simulink model "control"  (R2020a)
settings: Solver=FixedStepDiscrete  StartTime=0.0  StopTime=1  FixedStep=0.0005  RelTol=1e-3  EnableMultiTasking=on
undefined symbols (not defined in the file): acc_calmax1, acc_calmax2, acc_calmin1, acc_calmin2, akemancanshu, bre, bre_calmax, bre_calmin, ecucoder_acal, I_AN01_5K1, I_AN03_5V, I_AN04_5V, kd, ki, kp, leftmax, O_SW06_HS1A, rightmax, T_add, T_del, tiaoshi, zhiling
libraries: ec5744lib x252, canmsglib x92, simulink x5
(part 7 of 9)

== system control/Subsystem/run/analog_input/无人意图转译/无人/Subsystem1/Desired ==
  此处输入感知的期望整车纵向速度 : Inport
  输入整车加速度测量值1 : Inport  Port=2
  输入整车车速测量值1 : Inport  Port=3
  Data Store Read3 : DataStoreRead  DataStoreName=match_model
  Data Store Write : DataStoreWrite  Commented=on  DataStoreName=acc
  MATLAB Function : MATLAB Function  TreatAsAtomicUnit=on
  MATLAB Function1 : MATLAB Function  Commented=on  TreatAsAtomicUnit=on
  MATLAB Function2 : MATLAB Function  TreatAsAtomicUnit=on
  Subsystem : Subsystem
  Subsystem1 : Subsystem
  ddotx1d输入1 : Outport
  dotx1d输入 : Outport  Port=2
  x1d输入 : Outport  Port=3
  输入整车加速度测量值x2 : Outport  Port=4
  输入整车车速测量值x1 : Outport  Port=5
  wires:
  此处输入感知的期望整车纵向速度/1 -> MATLAB Function2/7(v1), Subsystem1/1(y), MATLAB Function/1(u)
  输入整车加速度测量值1/1 -> 输入整车加速度测量值x2/1
  MATLAB Function1/1(y) -> ddotx1d输入1/1
  MATLAB Function/1(y) -> MATLAB Function2/1(u1), Subsystem/1(y)
  MATLAB Function2/1(y) -> MATLAB Function1/1(u), dotx1d输入/1, Data Store Write/1
  Subsystem/1(u2) -> MATLAB Function2/2(u2)
  Subsystem/2(u3) -> MATLAB Function2/3(u3)
  Subsystem/3(u4) -> MATLAB Function2/4(u4)
  Subsystem/4(u5) -> MATLAB Function2/5(u5)
  输入整车车速测量值1/1 -> 输入整车车速测量值x1/1
  Data Store Read3/1 -> MATLAB Function2/6(model)
  Subsystem1/1(u2) -> MATLAB Function2/8(v2)
  Subsystem1/2(u3) -> MATLAB Function2/9(v3)
  Subsystem1/3(u4) -> MATLAB Function2/10(v4)
  Subsystem1/4(u5) -> MATLAB Function2/11(v5)
  MATLAB Function2/2(V) -> x1d输入/1

== system control/Subsystem/run/analog_input/无人意图转译/无人/Subsystem1/Subsystem ==
  note: 反馈系数，得调一下
  期望加速度（负值） : Inport
  x1d输入 : Inport  Port=2
  输入整车车速测量值x1 : Inport  Port=3
  Abs : Abs
  Abs1 : Abs
  MATLAB Function : MATLAB Function  TreatAsAtomicUnit=on
  Product : Product
  Sum : Sum  Inputs=|++
  pid_function : Subsystem
  整车质量 : Constant  Value=246
  总制动力 : Outport
  wires:
  期望加速度（负值）/1 -> pid_function/2(期望加速度（负值）), Abs/1
  Abs/1 -> Product/2
  整车质量/1 -> Product/1
  Product/1 -> Sum/1
  [A] -> pid_function/1(u)
  pid_function/1(output) -> Abs1/1
  Abs1/1 -> Sum/2
  Sum/1 -> MATLAB Function/1(u)
  输入整车车速测量值x1/1 -> MATLAB Function/2(v)
  x1d输入/1 -> MATLAB Function/3(vd)
  MATLAB Function/1(y) -> 总制动力/1

== system control/Subsystem/run/analog_input/无人意图转译/无人/Subsystem1/计算四轮各自制动力 ==
  u : Inport
  Data Store Read : DataStoreRead  DataStoreName=M_expire
  MATLAB Function : MATLAB Function  TreatAsAtomicUnit=on
  输出左前的制动力 : Outport
  输出右前的制动力2 : Outport  Port=2
  输出左后轮的制动力3 : Outport  Port=3
  输出右后轮的制动力1 : Outport  Port=4
  wires:
  u/1 -> MATLAB Function/1(u)
  MATLAB Function/1(y1) -> 输出左前的制动力/1
  MATLAB Function/2(y2) -> 输出右前的制动力2/1
  MATLAB Function/3(y3) -> 输出左后轮的制动力3/1
  MATLAB Function/4(y4) -> 输出右后轮的制动力1/1
  Data Store Read/1 -> MATLAB Function/2(deltaM)

== system control/Subsystem/run/ctrl/Subsystem1/control_strategy/Subsystem/Rules ==
  as : Inport
  am : Inport  Port=2
  ab : Inport  Port=3
  bnb : Inport  Port=4
  bns : Inport  Port=5
  bo : Inport  Port=6
  bps : Inport  Port=7
  bpb : Inport  Port=8
  DNB : MinMax  Function=max
  DNS : MinMax  Function=max  Inputs=3
  DO : MinMax  Function=max  Inputs=3
  DPB : MinMax  Function=max  Inputs=4
  DPS : MinMax  Function=max  Inputs=4
  Min(AB,BNB) : MinMax  Inputs=2
  Min(AB,BNS) : MinMax  Inputs=2
  Min(AB,BO) : MinMax  Inputs=2
  Min(AB,BPB) : MinMax  Inputs=2
  Min(AB,BPS) : MinMax  Inputs=2
  Min(AM,BNB) : MinMax  Inputs=2
  Min(AM,BNS) : MinMax  Inputs=2
  Min(AM,BO) : MinMax  Inputs=2
  Min(AM,BPB) : MinMax  Inputs=2
  Min(AM,BPS) : MinMax  Inputs=2
  Min(AS,BNB) : MinMax  Inputs=2
  Min(AS,BNS) : MinMax  Inputs=2
  Min(AS,BO) : MinMax  Inputs=2
  Min(AS,BPB) : MinMax  Inputs=2
  Min(AS,BPS) : MinMax  Inputs=2
  dnb : Outport  VectorParamsAs1DForOutWhenUnconnected=off
  dns : Outport  Port=2  VectorParamsAs1DForOutWhenUnconnected=off
  do : Outport  Port=3  VectorParamsAs1DForOutWhenUnconnected=off
  dps : Outport  Port=4  VectorParamsAs1DForOutWhenUnconnected=off
  dpb : Outport  Port=5  VectorParamsAs1DForOutWhenUnconnected=off
  wires:
  Min(AS,BNS)/1 -> DNS/1
  Min(AB,BNB)/1 -> DNS/3
  bps/1 -> Min(AB,BPS)/2, Min(AM,BPS)/2, Min(AS,BPS)/2
  bo/1 -> Min(AB,BO)/2, Min(AM,BO)/2, Min(AS,BO)/2
  bpb/1 -> Min(AB,BPB)/2, Min(AM,BPB)/2, Min(AS,BPB)/2
  as/1 -> Min(AS,BPB)/1, Min(AS,BPS)/1, Min(AS,BO)/1, Min(AS,BNS)/1, Min(AS,BNB)/1
  Min(AS,BNB)/1 -> DNB/1
  Min(AS,BPB)/1 -> DPB/1
  bns/1 -> Min(AB,BNS)/2, Min(AM,BNS)/2, Min(AS,BNS)/2
  Min(AB,BNS)/1 -> DO/3
  ab/1 -> Min(AB,BPB)/1, Min(AB,BPS)/1, Min(AB,BO)/1, Min(AB,BNS)/1, Min(AB,BNB)/1
  bnb/1 -> Min(AM,BNB)/2, Min(AS,BNB)/2, Min(AB,BNB)/2
  Min(AM,BO)/1 -> DPS/3
  am/1 -> Min(AM,BPB)/1, Min(AM,BPS)/1, Min(AM,BO)/1, Min(AM,BNS)/1, Min(AM,BNB)/1
  Min(AB,BPB)/1 -> DPB/3
  Min(AM,BNB)/1 -> DNS/2
  Min(AS,BPS)/1 -> DPS/1
  Min(AM,BPS)/1 -> DPS/2
  Min(AM,BNS)/1 -> DO/2
  Min(AB,BO)/1 -> DPS/4
  Min(AS,BO)/1 -> DO/1
  Min(AM,BPB)/1 -> DPB/2
  Min(AB,BPS)/1 -> DPB/4
  DO/1 -> do/1
  DNB/1 -> dnb/1
  DNS/1 -> dns/1
  DPS/1 -> dps/1
  DPB/1 -> dpb/1

== system control/Subsystem/run/ctrl/Subsystem1/control_strategy/差速/差速 ==
  note: *待更改
  Data Store Read : DataStoreRead  DataStoreName=workstation_steering
  Data Store Read1 : DataStoreRead  DataStoreName=V_Kalman
  Data Store Read2 : DataStoreRead  DataStoreName=A_cexiang
  Data Store Read3 : DataStoreRead  DataStoreName=ACC_Z
  Data Store Read4 : DataStoreRead  Commented=on  DataStoreName=dianji_velcoity_zuoqian
  Data Store Read5 : DataStoreRead  Commented=on  DataStoreName=dianji_velcoity_youqian
  Data Store Read6 : DataStoreRead  Commented=on  DataStoreName=dianji_velcoity_zuohou
  Data Store Read7 : DataStoreRead  Commented=on  DataStoreName=dianji_velcoity_youhou
  Data Store Read8 : DataStoreRead  DataStoreName=workstation_steering
  Data Store Write1 : DataStoreWrite  Commented=on  DataStoreName=Vzuoqian
  Data Store Write2 : DataStoreWrite  Commented=on  DataStoreName=Vyouqian
  Data Store Write3 : DataStoreWrite  Commented=on  DataStoreName=Vzuohou
  Data Store Write4 : DataStoreWrite  Commented=on  DataStoreName=Vyouhou
  LQR差速 : MATLAB Function  TreatAsAtomicUnit=on
  MATLAB Function : MATLAB Function  TreatAsAtomicUnit=on
  Product : Product
  Sum : Sum  Inputs=|+-
  pid : MATLAB Function  Commented=on  TreatAsAtomicUnit=on
  pid1 : MATLAB Function  Commented=on  TreatAsAtomicUnit=on
  pid2 : MATLAB Function  Commented=on  TreatAsAtomicUnit=on
  pid3 : MATLAB Function  Commented=on  TreatAsAtomicUnit=on
  期望横摆力矩计算 : MATLAB Function  TreatAsAtomicUnit=on
  转动惯量 : Constant  Value=145
  阿克曼转向 : MATLAB Function  Commented=on  TreatAsAtomicUnit=on
  M : Outport
  wires:
  Product/1 -> Sum/2
  MATLAB Function/1(y) -> 期望横摆力矩计算/1(delta)
  期望横摆力矩计算/1(Mz) -> Sum/1
  Data Store Read1/1 -> 阿克曼转向/1(v), 期望横摆力矩计算/2(Vx)
  转动惯量/1 -> Product/1, LQR差速/3(J)
  Data Store Read/1 -> MATLAB Function/1(u)
  Sum/1 -> LQR差速/1(yaw_error)
  Data Store Read3/1 -> Product/2, LQR差速/2(yaw_rate)
  阿克曼转向/3(wrl) -> Data Store Write3/1
  Data Store Read4/1 -> pid/1(v)
  Data Store Read7/1 -> pid3/1(v)
  阿克曼转向/2(wfr) -> Data Store Write2/1
  Data Store Read5/1 -> pid1/1(v)
  Data Store Read2/1 -> 阿克曼转向/2(a), 期望横摆力矩计算/3(ax)
  阿克曼转向/1(wfl) -> Data Store Write1/1
  Data Store Read6/1 -> pid2/1(v)
  阿克曼转向/4(wrr) -> Data Store Write4/1
  Data Store Read8/1 -> 阿克曼转向/3(angle)
  LQR差速/1(M) -> M/1

== system control/Subsystem/run/ctrl/Subsystem1/control_strategy/限滑/MPC ==
  右后in : Inport
  左后in : Inport  Port=2
  右前in : Inport  Port=3
  左前in : Inport  Port=4
  MPC : Subsystem
  右后 : Outport
  左后 : Outport  Port=2
  右前 : Outport  Port=3
  左前 : Outport  Port=4
  wires:
  右后in/1 -> MPC/1(U_init)
  左后in/1 -> MPC/2(U_init1)
  右前in/1 -> MPC/3(U_init2)
  左前in/1 -> MPC/4(U_init3)
  MPC/1(右后) -> 右后/1
  MPC/2(左后) -> 左后/1
  MPC/3(右前) -> 右前/1
  MPC/4(左前) -> 左前/1

== system control/Subsystem/run/ctrl/Subsystem1/control_strategy/限滑/PID限滑 ==
  u : Inport
  Constant{,1..3} (4 alike) : Constant  Value=0.9
  Data Store Read : DataStoreRead  DataStoreName=slipyouhou
  Data Store Read1 : DataStoreRead  DataStoreName=slipyuoqian
  Data Store Read2 : DataStoreRead  DataStoreName=slipzuohou
  Data Store Read3 : DataStoreRead  DataStoreName=slipzuoqian
  Data Store Write : DataStoreWrite  DataStoreName=brake_slipyouhou
  Data Store Write1 : DataStoreWrite  DataStoreName=brake_slipzuohou
  Data Store Write2 : DataStoreWrite  DataStoreName=brake_slipzuoqian
  Data Store Write3 : DataStoreWrite  DataStoreName=brake_slipyouqian
  pid限滑与ABS : MATLAB Function  TreatAsAtomicUnit=on
  pid限滑与ABS1 : MATLAB Function  TreatAsAtomicUnit=on
  pid限滑与ABS2 : MATLAB Function  TreatAsAtomicUnit=on
  pid限滑与ABS3 : MATLAB Function  TreatAsAtomicUnit=on
  计算油压 : MATLAB Function  TreatAsAtomicUnit=on
  throttle_youhou : Outport
  throttle_youqian : Outport  Port=2
  throttle_zuohou : Outport  Port=3
  throttle_zuoqian : Outport  Port=4
  wires:
  Data Store Read/1 -> pid限滑与ABS/1(slip)
  Constant/1 -> pid限滑与ABS/2(slip_ratio_limit)
  Data Store Read2/1 -> pid限滑与ABS2/1(slip)
  Constant1/1 -> pid限滑与ABS1/2(slip_ratio_limit)
  Data Store Read3/1 -> pid限滑与ABS3/1(slip)
  pid限滑与ABS/1(throttle) -> throttle_youhou/1
  Constant3/1 -> pid限滑与ABS3/2(slip_ratio_limit)
  Data Store Read1/1 -> pid限滑与ABS1/1(slip)
  Constant2/1 -> pid限滑与ABS2/2(slip_ratio_limit)
  pid限滑与ABS3/1(throttle) -> throttle_zuoqian/1
  pid限滑与ABS1/1(throttle) -> throttle_youqian/1
  pid限滑与ABS2/1(throttle) -> throttle_zuohou/1
  pid限滑与ABS3/2(brake) -> 计算油压/1(y1)
  pid限滑与ABS1/2(brake) -> 计算油压/2(y2)
  pid限滑与ABS2/2(brake) -> 计算油压/3(y3)
  pid限滑与ABS/2(brake) -> 计算油压/4(y4)
  计算油压/4(p4) -> Data Store Write/1
  计算油压/1(p1) -> Data Store Write2/1
  计算油压/2(p2) -> Data Store Write3/1
  计算油压/3(p3) -> Data Store Write1/1
  u/1 -> pid限滑与ABS3/3(u), pid限滑与ABS2/3(u), pid限滑与ABS1/3(u), pid限滑与ABS/3(u)

== system control/Subsystem/run/ctrl/Subsystem1/control_strategy/限滑/Subsystem1 ==
  TP : Inport
  右后 : Inport  Port=2
  throttle_youhou : Inport  Port=3
  In4 : Inport  Port=4
  右前 : Inport  Port=5
  throttle_youqian : Inport  Port=6
  u : Inport  Port=7
  mpc : Inport  Port=8
  pid : Inport  Port=9
  In7 : Inport  Port=10
  左前 : Inport  Port=11
  throttle_zuoqian : Inport  Port=12
  Data Store Read : DataStoreRead  DataStoreName=slipyouhou
  Data Store Read1 : DataStoreRead  DataStoreName=slipyuoqian
  Data Store Read2 : DataStoreRead  DataStoreName=slipzuohou
  Data Store Read3 : DataStoreRead  DataStoreName=slipzuoqian
  Data Store Read4 : DataStoreRead  DataStoreName=match_model
  MATLAB Function2 : MATLAB Function  TreatAsAtomicUnit=on
  MATLAB Function3 : MATLAB Function  TreatAsAtomicUnit=on
  MATLAB Function4 : MATLAB Function  TreatAsAtomicUnit=on
  MATLAB Function5 : MATLAB Function  TreatAsAtomicUnit=on
  youhou : Outport
  youqian : Outport  Port=2
  zuohou : Outport  Port=3
  zuoqian : Outport  Port=4
  wires:
  pid/1 -> MATLAB Function5/3(pid)
  mpc/1 -> MATLAB Function5/2(mpc)
  u/1 -> MATLAB Function5/1(u)
  In4/1 -> MATLAB Function4/1(u)
  右前/1 -> MATLAB Function4/2(mpc)
  throttle_youqian/1 -> MATLAB Function4/3(pid)
  throttle_youhou/1 -> MATLAB Function3/3(pid)
  右后/1 -> MATLAB Function3/2(mpc)
  TP/1 -> MATLAB Function3/1(u)
  throttle_zuoqian/1 -> MATLAB Function2/3(pid)
  左前/1 -> MATLAB Function2/2(mpc)
  In7/1 -> MATLAB Function2/1(u)
  Data Store Read/1 -> MATLAB Function3/4(slip)
  Data Store Read1/1 -> MATLAB Function4/4(slip)
  Data Store Read2/1 -> MATLAB Function5/4(slip)
  Data Store Read3/1 -> MATLAB Function2/4(slip)
  MATLAB Function3/1(y) -> youhou/1
  MATLAB Function2/1(y) -> zuoqian/1
  MATLAB Function5/1(y) -> zuohou/1
  MATLAB Function4/1(y) -> youqian/1
  Data Store Read4/1 -> MATLAB Function2/5(model), MATLAB Function5/5(model), MATLAB Function4/5(model), MATLAB Function3/5(model)

== system control/Subsystem/run/analog_input/无人意图转译/无人/Subsystem1/Desired/Subsystem ==
  y : Inport
  Delay : Delay  DelayLength=1
  Delay1 : Delay
  Delay2 : Delay  DelayLength=3
  Delay3 : Delay  DelayLength=4
  u2 : Outport
  u3 : Outport  Port=2
  u4 : Outport  Port=3
  u5 : Outport  Port=4
  wires:
  y/1 -> Delay3/1, Delay2/1, Delay1/1, Delay/1
  Delay/1 -> u2/1
  Delay1/1 -> u3/1
  Delay3/1 -> u5/1
  Delay2/1 -> u4/1

== system control/Subsystem/run/analog_input/无人意图转译/无人/Subsystem1/Desired/Subsystem1 ==
  y : Inport
  Delay : Delay  DelayLength=1
  Delay1 : Delay
  Delay2 : Delay  DelayLength=3
  Delay3 : Delay  DelayLength=4
  u2 : Outport
  u3 : Outport  Port=2
  u4 : Outport  Port=3
  u5 : Outport  Port=4
  wires:
  y/1 -> Delay3/1, Delay2/1, Delay1/1, Delay/1
  Delay/1 -> u2/1
  Delay1/1 -> u3/1
  Delay3/1 -> u5/1
  Delay2/1 -> u4/1

== system control/Subsystem/run/analog_input/无人意图转译/无人/Subsystem1/Subsystem/pid_function ==
  u : Inport
  期望加速度（负值） : Inport  Port=2
  Abs1 : Abs  Commented=on
  Gain : Gain  Commented=on
  Gain2 : Gain  Commented=on
  Subsystem : Subsystem  Commented=on
  integral : MATLAB Function  TreatAsAtomicUnit=on
  output : Outport
  wires:
  integral/1(output) -> output/1
  Gain/1 -> Abs1/1
  u/1 -> integral/1(u)
  Gain2/1 -> Subsystem/1(In1)
  期望加速度（负值）/1 -> integral/2(a)

== system control/Subsystem/run/ctrl/Subsystem1/control_strategy/限滑/MPC/MPC ==
  U_init : Inport
  U_init1 : Inport  Port=2
  U_init2 : Inport  Port=3
  U_init3 : Inport  Port=4
  Data Store Read : DataStoreRead  DataStoreName=slipyouhou
  Data Store Read1 : DataStoreRead  DataStoreName=slipzuohou
  Data Store Read2 : DataStoreRead  DataStoreName=slipyuoqian
  Data Store Read3 : DataStoreRead  DataStoreName=slipzuoqian
  MATLAB Function : MATLAB Function  TreatAsAtomicUnit=on
  MATLAB Function1 : MATLAB Function  TreatAsAtomicUnit=on
  MATLAB Function2 : MATLAB Function  TreatAsAtomicUnit=on
  MATLAB Function3 : MATLAB Function  TreatAsAtomicUnit=on
  MPC右前 : Subsystem
  MPC右后 : Subsystem
  MPC左前 : Subsystem
  MPC左后 : Subsystem
  右后 : Outport
  左后 : Outport  Port=2
  右前 : Outport  Port=3
  左前 : Outport  Port=4
  wires:
  MPC右前/1(右前) -> 右前/1
  MPC左前/1(左前) -> 左前/1
  MPC右后/1(右后) -> 右后/1
  U_init3/1 -> MPC左前/1(U_init)
  MPC左后/1(左后) -> 左后/1
  U_init1/1 -> MPC左后/1(U_init)
  U_init2/1 -> MPC右前/1(U_init)
  U_init/1 -> MPC右后/1(U_init)
  Data Store Read/1 -> MATLAB Function/1(u)
  MATLAB Function/1(y) -> MPC右后/Enable
  Data Store Read1/1 -> MATLAB Function1/1(u)
  MATLAB Function1/1(y) -> MPC左后/Enable
  Data Store Read2/1 -> MATLAB Function2/1(u)
  MATLAB Function2/1(y) -> MPC右前/Enable
  Data Store Read3/1 -> MATLAB Function3/1(u)
  MATLAB Function3/1(y) -> MPC左前/Enable

== system control/Subsystem/run/analog_input/无人意图转译/无人/Subsystem1/Subsystem/pid_function/Subsystem ==
  In1 : Inport
  Constant1 : Constant  Value=0.02
  Delay1 : Delay  DelayLength=1
  Divide1 : Product  Inputs=*/
  Sum4 : Sum  Inputs=|+-
  Out1 : Outport
  wires:
  Divide1/1 -> Out1/1
  Constant1/1 -> Divide1/2
  Sum4/1 -> Divide1/1
  Delay1/1 -> Sum4/2
  In1/1 -> Sum4/1, Delay1/1

== system control/Subsystem/run/ctrl/Subsystem1/control_strategy/限滑/MPC/MPC/MPC右前 ==
  U_init : Inport
  Enable : EnablePort
  Constant : Constant  Value=0.17
  Data Store Read : DataStoreRead  DataStoreName=slipyuoqian
  MPC_function : MATLAB Function  TreatAsAtomicUnit=on
  Sum : Sum  Inputs=|+-
  右前 : Outport
  wires:
  Data Store Read/1 -> Sum/1
  Constant/1 -> Sum/2
  MPC_function/1(u_k) -> 右前/1
  Sum/1 -> MPC_function/1(x_k)
  U_init/1 -> MPC_function/2(U_init)

== system control/Subsystem/run/ctrl/Subsystem1/control_strategy/限滑/MPC/MPC/MPC右后 ==
  U_init : Inport
  Enable : EnablePort
  Constant : Constant  Value=0.17
  Data Store Read : DataStoreRead  DataStoreName=slipyouhou
  MPC_function : MATLAB Function  TreatAsAtomicUnit=on
  Sum : Sum  Inputs=|+-
  右后 : Outport
  wires:
  Data Store Read/1 -> Sum/1
  Constant/1 -> Sum/2
  MPC_function/1(u_k) -> 右后/1
  Sum/1 -> MPC_function/1(x_k)
  U_init/1 -> MPC_function/2(U_init)

== system control/Subsystem/run/ctrl/Subsystem1/control_strategy/限滑/MPC/MPC/MPC左前 ==
  U_init : Inport
  Enable : EnablePort
  Constant : Constant  Value=0.17
  Data Store Read : DataStoreRead  DataStoreName=slipzuoqian
  MPC_function : MATLAB Function  TreatAsAtomicUnit=on
  Sum : Sum  Inputs=|+-
  左前 : Outport
  wires:
  Data Store Read/1 -> Sum/1
  Constant/1 -> Sum/2
  MPC_function/1(u_k) -> 左前/1
  Sum/1 -> MPC_function/1(x_k)
  U_init/1 -> MPC_function/2(U_init)

== system control/Subsystem/run/ctrl/Subsystem1/control_strategy/限滑/MPC/MPC/MPC左后 ==
  U_init : Inport
  Enable : EnablePort
  Constant : Constant  Value=0.17
  Data Store Read : DataStoreRead  DataStoreName=slipzuohou
  MPC_function : MATLAB Function  TreatAsAtomicUnit=on
  Sum : Sum  Inputs=|+-
  左后 : Outport
  wires:
  Data Store Read/1 -> Sum/1
  Constant/1 -> Sum/2
  MPC_function/1(u_k) -> 左后/1
  Sum/1 -> MPC_function/1(x_k)
  U_init/1 -> MPC_function/2(U_init)

== matlab function control/Subsystem/run/analog_input/有人/Subsystem/MATLAB Function2 ==
  data: u input; y output; min input; max input
function y = fcn(u,min,max)

y = (double(u)-min-4640)/(-min+max-4640+4550);

== matlab function control/Subsystem/Tx/TX控制器/速度/188右后/MATLAB Function ==
  data: u input; y output; zhidongesc input; zhidongebs input
function y = fcn(u,zhidongesc,zhidongebs)
 y = u*594.06;
if zhidongesc>1800&&zhidongebs==2
    y = u*594.06;
end
if zhidongesc<1500&&zhidongebs==2
    y=0;
end

== matlab function control/Subsystem/Tx/TX控制器/速度/188右后/MATLAB Function3 ==
  data: v input; y output; angle input; vz input; model input
function y = fcn(v, angle,vz,model)
if (angle>3||angle<-3)&&model==3%4650000,4870000,4741002
    y=vz*594.06;
else
    y = v;
end

== matlab function control/Subsystem/Tx/TX控制器/速度/189左后/MATLAB Function3 ==
  data: v input; y output; angle input; vz input; model input
function y = fcn(v, angle, vz,model)
if (angle>3||angle<-3)&&model==3%4650000,4870000,4741002
    y=vz*594.06;
else
    y = v;
end

== matlab function control/Subsystem/Tx/转向/转向换算/Subsystem/MATLAB Function1 ==
  data: u input; y output
function y = fcn(u)

y = (u-2.846e+04)/3255;

== matlab function control/Subsystem/Tx/TX控制器/Subsystem1/MATLAB Function2 ==
  data: anglenb input; youqianvvv output; v input; zuoqianvvv output; youhouvvv output; zuohouvvv output; model input; k input
function [youqianvvv,zuoqianvvv,youhouvvv,zuohouvvv] = fcn(anglenb,v,model,k)

angle=anglenb*pi/180;
if model==3
    k=k+0.5;
    if angle>0
        zuohouvvv=v*(1.53/(k*angle)+1.16)/(1.53/(k*angle)+0.58);
        youhouvvv=v*(1.53/(k*angle))/(1.53/(k*angle)+0.58);
        zuoqianvvv=v*(1.53/(k*angle)+1.18)/(1.53/(k*angle)+0.59);
        youqianvvv=v*(1.53/(k*angle))/(1.53/(k*angle)+0.59);
    else
        youhouvvv=v*(1.53/(-k*angle)+1.16)/(-1.53/(k*angle)+0.58);
        zuohouvvv=v*(-1.53/(k*angle))/(-1.53/(k*angle)+0.58);
        youqianvvv=v*(-1.53/(k*angle)+1.18)/(-1.53/(k*angle)+0.59);
        zuoqianvvv=v*(-1.53/(k*angle))/(-1.53/(k*angle)+0.59);
    end
else
    zuohouvvv=v;
    youhouvvv=v;
    zuoqianvvv=v;
    youqianvvv=v;
end

== matlab function control/Subsystem/Tx/TX控制器/速度/188右后/MATLAB Function5 ==
  data: v input; y output; angle input; vz input; model input
function y = fcn(v, angle, vz,model)
if(angle>3||angle<-3)&&model==3%4650000,4870000,4741002
    y=vz*594.06;
else
    y = v;
end

== matlab function control/无人TX1/MATLAB Function1 ==
  data: model input; y output; status input
function y = fcn(model,status)
if (model==2)
    y=1;
else
    y=0;
end

== matlab function control/无人TX1/转向自动标定/MATLAB Function ==
  data: biaozhi1 output
function biaozhi1  = fcn()
persistent i;
     % 初始化状态变量
    if isempty(i)
        i = 1;
    end

    if i>4
        biaozhi1=1;
    else
        biaozhi1=0;       
    end
i=i+1;
end

== matlab function control/无人TX1/转向自动标定/MATLAB Function1 ==
  data: y1 output; y2 output; biaozhi2 output
function [y1,y2,biaozhi2] = fcn()
    persistent i;
     % 初始化状态变量
    if isempty(i)
        i = 1;
    end
    
    if i<4
        biaozhi2=1;
    else
        biaozhi2=0;
    end
    if mod(i, 2) == 0
        result = 1;
    else
        result = 0;
    end
    
    if result==0
        y1=6307883;
        y2=0;
    else
        y1=6307883;
        y2=128;
    end
    i=i+1;

== matlab function control/Subsystem/Tx/Toworkstation/MATLAB Function ==
  data: u input; y output
function y = fcn(u)
if u~=0&&u~=9&&u~=2
    y=1;
else
    y=0;
end

== matlab function control/Subsystem/Tx/esc，ABS/Subsystem/MATLAB Function ==
  data: u input; y output; status input
function y = fcn(u,status)
y = u;
if status==5
    u=4500;
end

== matlab function control/Subsystem/Tx/esc，ABS/Subsystem/MATLAB Function1 ==
  data: u input; y output; status input
function y = fcn(u,status)
y = u;
if status==5
    u=4500;
end

== matlab function control/Subsystem/Tx/esc，ABS/Subsystem/MATLAB Function2 ==
  data: u input; y output; status input
function y = fcn(u,status)
y = u;
if status==5
    u=4500;
end

== matlab function control/Subsystem/Tx/esc，ABS/Subsystem/MATLAB Function3 ==
  data: u input; y output; status input
function y = fcn(u,status)
y = u;
if status==5
    u=4500;
end

== matlab function control/无人TX1/转向自动标定/Subsystem/MATLAB Function ==
  data: steer output; y output; rm input; lm input; bianmaqi input; k output; d output
function [steer,y,k,d] = fcn(rm,lm,bianmaqi)
%使用前请将转向打到最左侧
lm=lm+3000;
rm=rm-3000;
k=0;
d=0;
  persistent i  A B;
     % 初始化状态变量
    if isempty(i)
        i = 0;
        A=zeros(120,1);
        B=zeros(120,1);
    end
 
    if i>20&&i<=140  
        j=i-20;
        delta=(rm-lm)/120;
        steer= lm+j*delta ;
        if (j>=1&&j<=120)
            B(j,1)=steer-delta;
            A(j,1)=bianmaqi;
        end
        
    else
      if i>=140
            N=length(A);
%             bb=0;
%             aa=0;
%             for l=1:120
%                 bbb=bb+B(l,1);
%                 aaa=aa+A(l,1);
%             end
%             bbar=bbb/120;
%             abar=aaa/120;
            k=(sum(B.*A)-N*mean(B)*mean(A))/(sum(A.^2)-N*mean(A)^2);
            d=mean(B)-k*mean(A);
%             steer=single(d);
        end
        steer=lm;
    end

    i=i+1;
  persistent time  a b;
     % 初始化状态变量
    if isempty(time)
        time = 0;
   
        a=5;
        b=10;
    end
    if mod(abs(time), 2) == 0
        result = 1;
    else
        result = 0;
    end
    if time<b&&result==0
    y=6;
 
    elseif time<b&&result==1
    y=15;
  
    elseif time>=b
        if result==1
            y=79;
        else
            y=63;
        end
    else
        y=6;
    end   
    time=time+1;
 
%     
%       persistent time1;
%      % 初始化状态变量
%     if isempty(time1)
%         time1 = 0;
%     end
%     if mod(time1, 2) == 0
%         result1 = 1;
%     else
%         result1 = 0;
%     end
%     if time1<2
%     y=6;
%  
%     elseif time1>=2&&time1<4
%     y=15;
%   
%     elseif time1>=4
%         if result1==1
%             y=79;
%         else
%             y=63;
%         end
%     else
%         y=6;
%     end   
%     time1=time1+1;
   
end

== matlab function control/Subsystem/run/analog_input/有人/Subsystem/踏板冲突 ==
  data: acc_fin_sig1 input; y output; acc_fin_sig2 input; bre_ori_sig input; bre input
function y = fcn(acc_fin_sig1, acc_fin_sig2,bre_ori_sig,bre)
if abs(acc_fin_sig1-acc_fin_sig2)> 2
    y=0;
elseif acc_fin_sig1>0.3&&bre_ori_sig+bre>=1
    y=0;
elseif acc_fin_sig1>5||acc_fin_sig2>5
    y=0;
else
    y=acc_fin_sig2;
end

== matlab function control/Subsystem/run/analog_input/有人/Subsystem/Subsystem1/MATLAB Function ==
  data: u input; y output
function y = fcn(u)
if u==0
    y=0;
else
    y=1;
end

== matlab function control/Subsystem/run/analog_input/有人/Subsystem1/MATLAB Function ==
  data: v input; T output
function T = fcn(v)
%#codegen
if v<6000*1.88e-3
    T=2100;
elseif v>11000*1.88e-3
    T=800;
else
    T=1100;
end

== matlab function control/Subsystem/Tx/TX控制器/速度/188右后/MATLAB Function6 ==
  data: v input; T output; a input
function T = fcn(v,a)
% if a>5
%     y = u;
% elseif a>3&&a<5
%     y=1200;
% else
%     y=800;
% end

if v<6000*1.88e-3
    T=2100;
elseif v>11000*1.88e-3
    T=800;
else
    T=1100;
end

== matlab function control/Subsystem/run/analog_input/有人/Subsystem1/MATLAB Function1 ==
  data: T input; TP output
function TP= fcn(T)
if T<10
    TP=0;
else
    TP=T;
end

== matlab function control/Subsystem/run/ctrl/Subsystem1/control_strategy/E,H ==
  data: A input; E output; B input; Q input; R input; F input; N input; H output; J output
function [E,H,J] = MPC_Matrices(A,B,Q,R,F,N)
    n=size(A,1); % A是n*n矩阵,得到n
    p=size(B,2); % B是n*p矩阵,得到p
    M=[eye(n);zeros(N*n,n)]; % 初始化M矩阵,M矩阵是(N+1)n*n的,
                             % 它上面是n*n个"I",这一步先把下半部分写成0
    C=zeros((N+1)*n,N*p); % 初始化C矩阵,这一步令它有(N+1)n*NP个0
     D=zeros(1,N*p);
    % 定义M和C
    tmp=eye(n); % 定义一个n*n 的 I 矩阵
    % 更新Ｍ和C
    for i=1:N % 循环,i从1到N
        rows =i*n+(1:n); %定义当前行数,从i*n开始，共n行
        C(rows,:)=[tmp*B,C(rows-n, 1:end-p)]; %将c矩阵填满
        tmp= A*tmp; %每一次将tmp左乘一次A
        M(rows,:)=tmp; %将M矩阵写满
    end
    % 定义Q_bar和R_bar
    Q_bar = kron(eye(N),Q);
    Q_bar = blkdiag(Q_bar,F);
    R_bar = kron(eye(N),R);
    % 计算G,E,H
    G=M'*Q_bar*M; % G: n*n
    E=C'*Q_bar*M; % E: NP*n
    H=C'*Q_bar*C+R_bar; % NP*NP
for i=1:N % 循环,i从1到N
     D(i)= 0.17;
end
  J=C'*Q_bar*D'

== matlab function control/Subsystem/run/ctrl/Subsystem1/control_strategy/MATLAB Function ==
  data: slip_ratio_fl input; torque_cmd_fl output; slip_ratio_fr input; slip_ratio_rl input; slip_ratio_rr input; desired_slip_ratio input; driver_torque_cmd_fl input; driver_torque_cmd_fr input; driver_torque_cmd_rl input; driver_torque_cmd_rr input; dt input; B input; C input; D input; E input; wheel_radius input; torque_cmd_fr output; torque_cmd_rl output; torque_cmd_rr output
function [torque_cmd_fl, torque_cmd_fr, torque_cmd_rl, torque_cmd_rr] = SlipRatioControlWithMagicFormula(slip_ratio_fl, slip_ratio_fr, slip_ratio_rl, slip_ratio_rr, desired_slip_ratio, driver_torque_cmd_fl, driver_torque_cmd_fr, driver_torque_cmd_rl, driver_torque_cmd_rr, dt, B, C, D, E, wheel_radius)

    % 定义持久变量来存储每个轮胎的上一次误差
    persistent e_prev_fl e_prev_fr e_prev_rl e_prev_rr
    if isempty(e_prev_fl)
        e_prev_fl = 0; e_prev_fr = 0; e_prev_rl = 0; e_prev_rr = 0;
    end

    % 滑膜设计参数
    lambda = 2;            
    K = 0.2;               
    delta = 0.05;          

    % 定义一个内部函数来为每个轮胎进行滑膜控制
    function [torque_cmd, e_prev] = singleWheelControl(slip_ratio, desired_slip_ratio, driver_torque_cmd, e_prev, B, C, D, E, wheel_radius)
        % 计算误差和误差的变化率
        e = desired_slip_ratio - slip_ratio;
        e_dot = (e - e_prev) / dt;
        s = e_dot + lambda * e;

        % 使用Magic Formula计算期望的轮胎纵向力
        Fx_desired = D * sin(C * atan(B * desired_slip_ratio - E*(B * desired_slip_ratio - atan(B * desired_slip_ratio))));
        
        % 转换纵向力为期望扭矩
        desired_torque = Fx_desired * wheel_radius;

        % 根据滑模控制策略调整扭矩
        if abs(s) < delta
            torque_adjustment = 0;
        else
            torque_adjustment = K * s;
        end

        % 结合Magic Formula期望扭矩和滑模控制调整来计算输出扭矩
        torque_cmd = desired_torque + torque_adjustment;
        
        % 保证输出扭矩为非负
        torque_cmd = max(0, torque_cmd); 

        % 更新误差以供下次使用
        e_prev = e;
    end

    % 为每个轮胎应用滑模控制策略
    [torque_cmd_fl, e_prev_fl] = singleWheelControl(slip_ratio_fl, desired_slip_ratio, driver_torque_cmd_fl, e_prev_fl, B, C, D, E, wheel_radius);
    [torque_cmd_fr, e_prev_fr] = singleWheelControl(slip_ratio_fr, desired_slip_ratio, driver_torque_cmd_fr, e_prev_fr, B, C, D, E, wheel_radius);
    [torque_cmd_rl, e_prev_rl] = singleWheelControl(slip_ratio_rl, desired_slip_ratio, driver_torque_cmd_rl, e_prev_rl, B, C, D, E, wheel_radius);
    [torque_cmd_rr, e_prev_rr] = singleWheelControl(slip_ratio_rr, desired_slip_ratio, driver_torque_cmd_rr, e_prev_rr, B, C, D, E, wheel_radius);

end

== matlab function control/Subsystem/run/ctrl/Subsystem1/control_strategy/MATLAB Function1 ==
  data: y output; angle input
function y = fcn(angle)
if angle>30||angle<-30%4650000,4870000,4741002
    y=1;
else
    y = 0;
end

== matlab function control/Subsystem/run/ctrl/Subsystem1/control_strategy/MATLAB Function2 ==
  data: A output; B output; Q output; R output; F output; N output; p output
function [A,B,Q,R,F,N,p] = fcn()
% 定义状态矩阵 A, n*n 矩阵
A = 0;
% 定义输入矩阵 B, n*p 矩阵
R=1;
FN=1;
K=6.89;
B = R/(FN*K);
p = size(B,2);
% 定义Q矩阵，n*n 矩阵
Q = 100;
% 定义F矩阵，n*n 矩阵
F = 100;
% 定义R矩阵，p*p 矩阵
R = 1;
%定义预测区间K
N = 5;

== matlab function control/Subsystem/run/ctrl/Subsystem1/control_strategy/MATLAB Function3 ==
  data: y output; angle input
function y = fcn(angle)
if angle>10||angle<-10%4650000,4870000,4741002
    y=1;
else
    y = 0;
end

== matlab function control/Subsystem/run/ctrl/Subsystem1/control_strategy/MPC ==
  data: X_K input; y output; Prediction input; A input; B input; Q input; R input; F input
function y = fcn(X_K,Prediction,A,B,Q,R,F)
    U_K(:,k) = Prediction;
    % 计算第k+1步时状态变量的值
%     X_K(:,k+1) = (A*X_K(:,k) + B*U_K(:,k))-0.17*A;
end

== matlab function control/Subsystem/Tx/TX控制器/速度/189左后/MATLAB Function2 ==
  data: enable input; enable_1 input; T input; TargetVelocity output; AMK_TorqueLimitPositive output; enable output; errorreset output; blnverteron output; CAN_dbcon output; v input
function [TargetVelocity,AMK_TorqueLimitPositive,enable,errorreset,blnverteron,CAN_dbcon]= fcn(enable,enable_1,T,v)
if (enable_1==0)
    TargetVelocity=0;
    enable=0;
    errorreset=1;
    blnverteron=0;
    CAN_dbcon=0;
    AMK_TorqueLimitPositive=0;
elseif (enable==0 && enable_1==1)
    TargetVelocity=2000;
    enable=1;
    errorreset=0;
    blnverteron=1;
    CAN_dbcon=1;
    AMK_TorqueLimitPositive=0;
elseif (enable==1 && enable_1==1)
    TargetVelocity=2000;
    enable=1;
    errorreset=0;
    blnverteron=1;
    CAN_dbcon=1;
    AMK_TorqueLimitPositive=T;
else
    TargetVelocity=0;
    enable=0;
    errorreset=1;
    blnverteron=0;
    CAN_dbcon=0;
    AMK_TorqueLimitPositive=0;
end

end

== matlab function control/Subsystem/run/ctrl/Subsystem1/control_strategy/Subsystem/defuzzification ==
  data: dnb input; delta output; dns input; do input; dps input; dpb input; d1 input; d2 input; d3 input
function delta = fcn(dnb,dns,do,dps,dpb, d1,d2,d3)
delta = dnb*d1/3 + dns*d1 + do*d2 + dps*d3 + dpb*(1-d3/3);
end

== matlab function control/Subsystem/run/ctrl/Subsystem1/control_strategy/Subsystem/α sets ==
  data: alpha input; as output; am output; ab output; a1 input; a2 input
function [as,am,ab] = fcn(alpha, a1, a2)
if alpha < a1
    as = 1-(alpha/a1);
    am = alpha/a1;
    ab = 0;
elseif alpha < a2
    as = 0; 
    am = 1-(alpha-a1)/(a2-a1);
    ab = (alpha-a1)/(a2-a1);
else
    as = 0;
    am = 0;
    ab = 1;
end

== matlab function control/Subsystem/run/ctrl/Subsystem1/control_strategy/Subsystem/β sets ==
  data: beta input; bnb output; bns output; bo output; b1 input; b2 input; bps output; bpb output; b3 input
function [bnb,bns,bo,bps,bpb] = fcn(beta, b1, b2, b3)
if beta < b1
    bnb = 1-(beta+1)/(b1+1);
    bns = (beta+1)/(b1+1);
    bo  = 0;
    bps = 0;
    bpb = 0;
elseif beta < b2
    bnb = 0; 
    bns = 1-(beta-b1)/(b2-b1);
    bo = (beta-b1)/(b2-b1);
    bps = 0;
    bpb = 0;
elseif beta < b3
    bnb = 0;
    bns = 0;
    bo  = 1-(beta-b2)/(b3-b2);
    bps = (beta-b2)/(b3-b2);
    bpb = 0;
else
    bnb = 0;
    bns = 0;
    bo  = 0;
    bps = 1-(beta-b3)/(1-b3);
    bpb = (beta-b3)/(1-b3);
end

== matlab function control/Subsystem/run/ctrl/Subsystem1/control_strategy/差速/MATLAB Function3 ==
  data: u input; youhou output; M input; youqian output; zuohou output; zuoqian output
function [youhou,youqian,zuohou,zuoqian] = fcn(u,M)
% U=4*u;
r=0.2032;%轮半径
B1=1.18;%左右轮距
B2=1.16;
youqian=M*r/(2*B2)+u;
youhou=youqian;
zuoqian=-M*r/(2*B1)+u;
zuohou=zuoqian;
end

== matlab function control/Subsystem/run/ctrl/Subsystem1/control_strategy/差速/差速/LQR差速 ==
  data: yaw_error input; M output; yaw_rate input; J input
% function M = carLQRControl(yaw_error, yaw_rate,J)
%     % 赛车LQR控制器参数
%     Q = diag([1, 1]); % 状态误差权重矩阵
%     R = 0.1; % 控制输入权重
%     
%     % 定义车辆模型参数
%     % J转动惯量
%     
%     % 设计LQR增益矩阵 K
%     A = [0, 1; 0, 0];%输入为期望与实际横摆力矩差值和横摆角速度
%     B = [0; J];
%     K = lqr(A, B, Q, R);
%     
%     % 计算横摆力矩控制输入
%     M = -K* [yaw_error; yaw_rate];
function M = carLQRControl(yaw_error, yaw_rate,J)
    % 赛车LQR控制器参数
    Q = diag([1, 1]); % 状态误差权重矩阵
    R = 0.1; % 控制输入权重
    
    % 设计LQR增益矩阵 K
    A = [0, 1; 0, 0]; % 输入为期望与实际横摆力矩差值和横摆角速度
    B = [0; J];
    
    % 使用迭代法求解代数Riccati方程，计算LQR增益矩阵 K
    max_iterations = 20;
    tolerance = 1e-2;
    P = eye(size(A));
%     for i = 1:max_iterations
%         P_new = Q + A' * P * A - A' * P * B * (R + B' * P * B)^(-1) * B' * P * A;
%         if max(abs(P_new - P), [], 'all') < tolerance
%             P = P_new;
%             break;
%         end
%         P = P_new;
%   K = (R + B' * P * B)^(-1) * B' * P * A;
%     end
     % 计算LQR增益矩阵 

 
   for k = 1:max_iterations
        F = inv(R+B'*P*B)*B'*P*A;
        P_new = (A-B*F)'*P*(A-B*F)+(F)'*R*(F)+Q;
        if max(abs(P_new - P), [], 'all') < tolerance
             P= P_new;
             F = inv(R+B'*P*B)*B'*P*A;
            break;
        end
        P= P_new;
    end
    F_N=F; 
   
    % 计算横摆力矩控制输入
    M = -F_N * [yaw_error; yaw_rate];

end

== matlab function control/Subsystem/run/ctrl/Subsystem1/control_strategy/差速/差速/MATLAB Function ==
  data: u input; y output
function y = fcn(u)

y = u;

== matlab function control/Subsystem/run/ctrl/Subsystem1/control_strategy/差速/差速/pid ==
  data: v input; u input; v_zuoqian output
function v_zuoqian  = carPIDControl(v, u)
    % 赛车PID控制器参数
    kp = 0.2;
    ki = 0.1;
    kd = 0.01;
    
    % 状态变量
    persistent integral previous_error 
    
    % 初始化状态变量
    if isempty(integral)
        integral = 0;
        previous_error = 0;
        i=0;
    end
    
    % PID控制器计算
    error = u - v;
    integral = integral + error*0.02;
    derivative = (error - previous_error)/0.02;
    
        if integral > 0.4    
        integral = 0.4;
        end
        if integral < -0.4    
        integral = -0.4;
        end
    
   v_zuoqian = kp * error + ki * integral + kd * derivative;
   
    % 保存上一个误差用于下次计算
    previous_error = error;
end

== matlab function control/Subsystem/run/ctrl/Subsystem1/control_strategy/差速/差速/pid1 ==
  data: v input; u input; v_zuoqian output
function v_zuoqian  = carPIDControl(v, u)
    % 赛车PID控制器参数
    kp = 0.2;
    ki = 0.1;
    kd = 0.01;
    
    % 状态变量
    persistent integral previous_error 
    
    % 初始化状态变量
    if isempty(integral)
        integral = 0;
        previous_error = 0;
        i=0;
    end
    
    % PID控制器计算
    error = u - v;
    integral = integral + error*0.02;
    derivative = (error - previous_error)/0.02;
    
        if integral > 0.4    
        integral = 0.4;
        end
        if integral < -0.4    
        integral = -0.4;
        end
    
   v_zuoqian = kp * error + ki * integral + kd * derivative;
   
    % 保存上一个误差用于下次计算
    previous_error = error;
end

== matlab function control/Subsystem/run/ctrl/Subsystem1/control_strategy/差速/差速/pid2 ==
  data: v input; u input; v_zuoqian output
function v_zuoqian  = carPIDControl(v, u)
    % 赛车PID控制器参数
    kp = 0.2;
    ki = 0.1;
    kd = 0.01;
    
    % 状态变量
    persistent integral previous_error 
    
    % 初始化状态变量
    if isempty(integral)
        integral = 0;
        previous_error = 0;
        i=0;
    end
    
    % PID控制器计算
    error = u - v;
    integral = integral + error*0.02;
    derivative = (error - previous_error)/0.02;
    
        if integral > 0.4    
        integral = 0.4;
        end
        if integral < -0.4    
        integral = -0.4;
        end
    
   v_zuoqian = kp * error + ki * integral + kd * derivative;
   
    % 保存上一个误差用于下次计算
    previous_error = error;
end

== matlab function control/Subsystem/run/ctrl/Subsystem1/control_strategy/差速/差速/pid3 ==
  data: v input; u input; v_zuoqian output
function v_zuoqian  = carPIDControl(v, u)
    % 赛车PID控制器参数
    kp = 0.2;
    ki = 0.1;
    kd = 0.01;
    
    % 状态变量
    persistent integral previous_error 
    
    % 初始化状态变量
    if isempty(integral)
        integral = 0;
        previous_error = 0;
        i=0;
    end
    
    % PID控制器计算
    error = u - v;
    integral = integral + error*0.02;
    derivative = (error - previous_error)/0.02;
    
        if integral > 0.4    
        integral = 0.4;
        end
        if integral < -0.4    
        integral = -0.4;
        end
    
   v_zuoqian = kp * error + ki * integral + kd * derivative;
   
    % 保存上一个误差用于下次计算
    previous_error = error;
end

== matlab function control/Subsystem/run/ctrl/Subsystem1/control_strategy/差速/差速/期望横摆力矩计算 ==
  data: delta input; Mz output; Vx input; ax input
function Mz = calculateYawMoment(delta,  Vx, ax)
    % 输入参数：
    % delta: 前轮转角 (rad)
    % Vx: 车辆速度 (m/s)
    % ax: 侧向加速度 (m/s^2)
    m=210;%: 车辆质量 (kg)
     lf=0.765;%: 前轴到重心的距离 (m)
     lr=0.765;%: 后轴到重心的距离 (m)
    
    % 轮胎侧向力估计，这里使用一个简化的线性模型
    Fy = ax * (lr * m * 9.81) / (lf + lr);
    delta=delta*pi/180
    % 计算期望的横摆力矩
    Mz = lf * Fy * cos(delta);
end

== matlab function control/Subsystem/run/ctrl/Subsystem1/control_strategy/差速/差速/阿克曼转向 ==
  data: wfl output; v input; wfr output; wrl output; wrr output; a input; angle input
function [wfl,wfr,wrl,wrr]= fcn(v,a,angle)
%22e轴距：1170mm 轮距 1530mm 前47%后53%即，前0.72后0.81 
L=1.53;%前后轴距    u是转角
d=1.17;%车宽
c1=0.93;%前车对角线的一半
c2=1;
k=1;%12.641传动比

Rcg=v^2/a;
if angle<0
    Rfr=sqrt(c1^2+Rcg^2-2*c1*Rcg*cos(2.25));
    Rfl=sqrt(c1^2+Rcg^2-2*c1*Rcg*cos(0.89));
    Rrl=sqrt(c2^2+Rcg^2-2*c2*Rcg*cos(0.945));
    Rrr=sqrt(c2^2+Rcg^2-2*c2*Rcg*cos(2.2));
    wfl=k*v/Rcg*Rfl;
    wfr=k*v/Rcg*Rfr;
    wrl=k*v/Rcg*Rrl;
    wrr=k*v/Rcg*Rrr;
else
    Rfl=sqrt(c1^2+Rcg^2-2*c1*Rcg*cos(2.25));
    Rfr=sqrt(c1^2+Rcg^2-2*c1*Rcg*cos(0.89));
    Rrr=sqrt(c2^2+Rcg^2-2*c2*Rcg*cos(0.945));
    Rrl=sqrt(c2^2+Rcg^2-2*c2*Rcg*cos(2.2));
    wfl=k*v/Rcg*Rfl;
    wfr=k*v/Rcg*Rfr;
    wrl=k*v/Rcg*Rrl;
    wrr=k*v/Rcg*Rrr; 
end
wfl=594.06*min(wfl,v+2);
wfr=594.06*min(wfr,v+2);
wrl=594.06*min(wrl,v+2);
wrr=594.06*min(wrr,v+2);
wfl=594.06*max(wfl,v-2);
wfr=594.06*max(wfr,v-2);
wrl=594.06*max(wrl,v-2);
wrr=594.06*max(wrr,v-2);

== matlab function control/Subsystem/run/ctrl/Subsystem1/control_strategy/滑模控制 ==
  data: slip_ratio_fl input; slip_ratio_fr input; slip_ratio_rl input; slip_ratio_rr input; torque_cmd_fl output; driver_torque_cmd_fl input; driver_torque_cmd_fr input; driver_torque_cmd_rl input; driver_torque_cmd_rr input; torque_cmd_fr output; torque_cmd_rl output; torque_cmd_rr output
function [torque_cmd_fl, torque_cmd_fr, torque_cmd_rl, torque_cmd_rr] = SlipRatioControl(slip_ratio_fl, slip_ratio_fr, slip_ratio_rl, slip_ratio_rr,   driver_torque_cmd_fl, driver_torque_cmd_fr, driver_torque_cmd_rl, driver_torque_cmd_rr)

    % 每个轮都有自己的误差历史记录
    persistent e_prev_fl e_prev_fr e_prev_rl e_prev_rr i driver_weight
    if isempty(e_prev_fl)
        e_prev_fl = 0; e_prev_fr = 0; e_prev_rl = 0; e_prev_rr = 0;
        driver_weight = 0.5;  % 车手命令的权重
        i=0;
    end

    % 设定参数
    lambda = 3;            % 滑模面设计参数
    K = 0.5;               % 滑模增益
    delta = 0.05;          % 滑模边界，小于此值时不做扭矩调整
%     driver_weight = 0.05;  % 车手命令的权重
    desired_slip_ratio=0.2;
    % 定义一个内部函数来进行滑膜控制，这样可以为每个轮重复使用
    function [torque_cmd, e_prev,e] = singleWheelControl(slip_ratio, desired_slip_ratio, driver_torque_cmd, e_prev)
        % 计算误差和误差的变化率
        e = desired_slip_ratio - slip_ratio;
        e_dot = (e - e_prev) / 0.02;
        s = e_dot + lambda * e;

        % 滑模控制策略
        if abs(s) < delta
            torque_adjustment = 0;  % s小于滑模边界时不做调整
        else
            torque_adjustment = K * s;  % 根据s的符号进行扭矩调整
        end

        % 结合车手的扭矩命令，并应用滑模控制的调整
        torque_cmd = driver_torque_cmd + driver_weight * driver_torque_cmd * torque_adjustment;
        torque_cmd = max(0, torque_cmd);  % 保证扭矩命令为正
        torque_cmd = min(2000, torque_cmd);  % 保证扭矩小于2000

        % 更新误差
        e_prev = e;
    end
    % 对每个轮应用滑模控制策略
    [torque_cmd_fl, e_prev_fl,efl] = singleWheelControl(slip_ratio_fl, desired_slip_ratio, driver_torque_cmd_fl, e_prev_fl);
    [torque_cmd_fr, e_prev_fr,efr] = singleWheelControl(slip_ratio_fr, desired_slip_ratio, driver_torque_cmd_fr, e_prev_fr);
    [torque_cmd_rl, e_prev_rl,erl] = singleWheelControl(slip_ratio_rl, desired_slip_ratio, driver_torque_cmd_rl, e_prev_rl);
    [torque_cmd_rr, e_prev_rr,err] = singleWheelControl(slip_ratio_rr, desired_slip_ratio, driver_torque_cmd_rr, e_prev_rr);
     %安全程序
     if (efl>0.8||efr>0.8||erl>0.8||err>0.8)
         i=i+1;
         if i>100
             driver_weight=0;
         end
     end
     if (efl<0.3&&efr<0.3&&erl<0.3&&err<0.3)
         i=0;
     end

end

== matlab function control/Subsystem/run/ctrl/Subsystem1/control_strategy/限滑/MATLAB Function ==
  data: slip_ratio_front_left input; torque_front_left output; slip_ratio_front_right input; slip_ratio_rear_left input; slip_ratio_rear_right input; e_prev input; dt input; torque_front_right output; torque_rear_left output; torque_rear_right output
function [torque_front_left, torque_front_right, torque_rear_left, torque_rear_right] = SlipRatioControl(slip_ratio_front_left, slip_ratio_front_right, slip_ratio_rear_left, slip_ratio_rear_right,  e_prev, dt)

% 参数设定
lambda = 5; % 调整因子，用于滑模面设计，实际应用中可能需要调整
boundary_thickness = 0.1; % 边界层厚度，用于sigmoid函数，以确保输出在合理范围内
max_torque = 2000; % 最大扭矩，表示车辆能够输出的最大扭矩
slip_ratio_desired=0.2;
% 内部函数，为每个轮子计算扭矩
function torque = computeTorque(slip_ratio_actual, e_prev)
    % 计算误差及其导数
    e = slip_ratio_desired - slip_ratio_actual;
    e_dot = (e - e_prev) / dt;
    
    % 滑模控制
    s = e_dot + lambda * e;
    
    % 使用软饱和函数（sigmoid函数）计算扭矩指令
    torque = max_torque / (1 + exp(-10 * (s - boundary_thickness)));
    
    % 限制扭矩值
    torque = min(max_torque, torque);
end

% 为每个轮子计算扭矩
torque_front_left = computeTorque(slip_ratio_front_left, e_prev(1));
torque_front_right = computeTorque(slip_ratio_front_right, e_prev(2));
torque_rear_left = computeTorque(slip_ratio_rear_left, e_prev(3));
torque_rear_right = computeTorque(slip_ratio_rear_right, e_prev(4));

% 更新上一次的误差
e_prev(1) = slip_ratio_desired - slip_ratio_front_left;
e_prev(2) = slip_ratio_desired - slip_ratio_front_right;
e_prev(3) = slip_ratio_desired - slip_ratio_rear_left;
e_prev(4) = slip_ratio_desired - slip_ratio_rear_right;

end

== matlab function control/Subsystem/Tx/TX控制器/速度/189左后/MATLAB Function4 ==
  data: u input; y output; zhidongesc input; zhidongebs input; huanting input
function y = fcn(u,zhidongesc,zhidongebs,huanting)
 y = u*594.06;
if zhidongesc>1800&&zhidongebs==2
    y = u*594.06;
end
if zhidongesc<1500&&zhidongebs==2
    y=0;
end
if huanting~=0
    y=0;
end

== matlab function control/Subsystem/run/ctrl/Subsystem1/control_strategy/限滑/MPC/MPC/MATLAB Function ==
  data: u input; y output
function y = fcn(u)
if u>=0.169&&u<=0.17
    y=1;
else
    y=0;
end

end

== matlab function control/Subsystem/run/ctrl/Subsystem1/control_strategy/限滑/MPC/MPC/MATLAB Function1 ==
  data: u input; y output
function y = fcn(u)
if u>=0.169&&u<=0.17
    y=1;
else
    y=0;
end

end

== matlab function control/Subsystem/run/ctrl/Subsystem1/control_strategy/限滑/MPC/MPC/MATLAB Function2 ==
  data: u input; y output
function y = fcn(u)

if u>=0.169&&u<=0.17
    y=1;
else
    y=0;
end

end

== matlab function control/Subsystem/run/ctrl/Subsystem1/control_strategy/限滑/MPC/MPC/MATLAB Function3 ==
  data: u input; y output
function y = fcn(u)

if u>=0.169&&u<=0.17
    y=1;
else
    y=0;
end

end

== matlab function control/Subsystem/run/ctrl/Subsystem1/control_strategy/限滑/MPC/MPC/MPC右前/MPC_function ==
  data: x_k input; u_k output; U_init input
function u_k= Prediction(x_k,U_init)
% 定义状态矩阵 A, n*n 矩阵
A = 0;
% 定义输入矩阵 B, n*p 矩阵
R=0.2032;
FN=2058;
K=6.89;
B = R/(FN*K);
p = size(B,2);
% 定义Q矩阵，n*n 矩阵
Q = 100;
% 定义F矩阵，n*n 矩阵
F = 100;
% 定义R矩阵，p*p 矩阵
R = 1;
% 定义迭代次数和学习率
maxIterations = 5;
learningRate = 0.3;
N=5;%预测区间
n=size(A,1); % A是n*n矩阵,得到n
p=size(B,2); % B是n*p矩阵,得到p
M=[eye(n);zeros(N*n,n)]; % 初始化M矩阵,M矩阵是(N+1)n*n的
D=[0.17;zeros(N*n,n)];
C=zeros((N+1)*n,N*p); % 初始化C矩阵,这一步令它有(N+1)n*NP个0

% 定义M和C
tmp=eye(n); % 定义一个n*n 的 I 矩阵
    for i=1:N % 循环,i从1到N
        rows =i*n+(1:n); %定义当前行数,从i*n开始，共n行
        C(rows,:)=[tmp*B,C(rows-n, 1:end-p)]; %将c矩阵填满
        tmp= A*tmp; %每一次将tmp左乘一次A
        M(rows,:)=tmp; %将M矩阵写满
         D(rows,:)=0.17;
    end
    % 定义Q_bar和R_bar
    Q_bar = kron(eye(N),Q);
    Q_bar = blkdiag(Q_bar,F);
    R_bar = kron(eye(N),R);
    % 计算G,E,H
    G=M'*Q_bar*M; % G: n*n
    E=C'*Q_bar*M; % E: NP*n
    H=C'*Q_bar*C+R_bar; % NP*NP
 J=(D'*Q_bar*C)';
 L=E*x_k+J;
 U = U_init*ones(N*p,1); % NP x 1
%  options = optimoptions('quadprog', 'Algorithm', 'active-set');
%  U_k = quadprog(H,L, [], [], [], [], 0*ones(5,1), 1100*ones(5,1), 100*ones(5,1), options);
    % 梯度下降法求解最优二次规划问题
    G=size(U,1);
    S=zeros(G*maxIterations,1);
    for i = 1:maxIterations
        % 计算目标函数的梯度
        gradient = 2*H*U + 2*L;
        % 更新变量 U，并保持在 [0, 1100] 范围内
        U = U - learningRate * gradient;
        U = max(U, 0);
        U = min(U, 1100);
        O=(i-1)*maxIterations+(1:maxIterations);
        S(O,1)=U;
    end

 u_k = S(1:p,1); % 取第一个结果
end

== matlab function control/Subsystem/run/ctrl/Subsystem1/control_strategy/限滑/MPC/MPC/MPC右后/MPC_function ==
  data: x_k input; u_k output; U_init input
function u_k= Prediction(x_k,U_init)
% 定义状态矩阵 A, n*n 矩阵
A = 0;
% 定义输入矩阵 B, n*p 矩阵
R=0.2032;
FN=2058;
K=6.89;
B = R/(FN*K);
p = size(B,2);
% 定义Q矩阵，n*n 矩阵
Q = 100;
% 定义F矩阵，n*n 矩阵
F = 100;
% 定义R矩阵，p*p 矩阵
R = 1;
% 定义迭代次数和学习率
maxIterations = 5;
learningRate = 0.3;
N=5;%预测区间
n=size(A,1); % A是n*n矩阵,得到n
p=size(B,2); % B是n*p矩阵,得到p
M=[eye(n);zeros(N*n,n)]; % 初始化M矩阵,M矩阵是(N+1)n*n的
D=[0.17;zeros(N*n,n)];
C=zeros((N+1)*n,N*p); % 初始化C矩阵,这一步令它有(N+1)n*NP个0

% 定义M和C
tmp=eye(n); % 定义一个n*n 的 I 矩阵
    for i=1:N % 循环,i从1到N
        rows =i*n+(1:n); %定义当前行数,从i*n开始，共n行
        C(rows,:)=[tmp*B,C(rows-n, 1:end-p)]; %将c矩阵填满
        tmp= A*tmp; %每一次将tmp左乘一次A
        M(rows,:)=tmp; %将M矩阵写满
         D(rows,:)=0.17;
    end
    % 定义Q_bar和R_bar
    Q_bar = kron(eye(N),Q);
    Q_bar = blkdiag(Q_bar,F);
    R_bar = kron(eye(N),R);
    % 计算G,E,H
    G=M'*Q_bar*M; % G: n*n
    E=C'*Q_bar*M; % E: NP*n
    H=C'*Q_bar*C+R_bar; % NP*NP
 J=(D'*Q_bar*C)';
 L=E*x_k+J;
 U = U_init*ones(N*p,1); % NP x 1
%  options = optimoptions('quadprog', 'Algorithm', 'active-set');
%  U_k = quadprog(H,L, [], [], [], [], 0*ones(5,1), 1100*ones(5,1), 100*ones(5,1), options);
    % 梯度下降法求解最优二次规划问题
    G=size(U,1);
    S=zeros(G*maxIterations,1);
    for i = 1:maxIterations
        % 计算目标函数的梯度
        gradient = 2*H*U + 2*L;
        % 更新变量 U，并保持在 [0, 1100] 范围内
        U = U - learningRate * gradient;
        U = max(U, 0);
        U = min(U, 1100);
        O=(i-1)*maxIterations+(1:maxIterations);
        S(O,1)=U;
    end

 u_k = S(1:p,1); % 取第一个结果
end

== matlab function control/Subsystem/run/ctrl/Subsystem1/control_strategy/限滑/MPC/MPC/MPC左前/MPC_function ==
  data: x_k input; u_k output; U_init input
function u_k= Prediction(x_k,U_init)
% 定义状态矩阵 A, n*n 矩阵
A = 0;
% 定义输入矩阵 B, n*p 矩阵
R=0.2032;
FN=2058;
K=6.89;
B = R/(FN*K);
p = size(B,2);
% 定义Q矩阵，n*n 矩阵
Q = 100;
% 定义F矩阵，n*n 矩阵
F = 100;
% 定义R矩阵，p*p 矩阵
R = 1;
% 定义迭代次数和学习率
maxIterations = 5;
learningRate = 0.3;
N=5;%预测区间
n=size(A,1); % A是n*n矩阵,得到n
p=size(B,2); % B是n*p矩阵,得到p
M=[eye(n);zeros(N*n,n)]; % 初始化M矩阵,M矩阵是(N+1)n*n的
D=[0.17;zeros(N*n,n)];
C=zeros((N+1)*n,N*p); % 初始化C矩阵,这一步令它有(N+1)n*NP个0

% 定义M和C
tmp=eye(n); % 定义一个n*n 的 I 矩阵
    for i=1:N % 循环,i从1到N
        rows =i*n+(1:n); %定义当前行数,从i*n开始，共n行
        C(rows,:)=[tmp*B,C(rows-n, 1:end-p)]; %将c矩阵填满
        tmp= A*tmp; %每一次将tmp左乘一次A
        M(rows,:)=tmp; %将M矩阵写满
         D(rows,:)=0.17;
    end
    % 定义Q_bar和R_bar
    Q_bar = kron(eye(N),Q);
    Q_bar = blkdiag(Q_bar,F);
    R_bar = kron(eye(N),R);
    % 计算G,E,H
    G=M'*Q_bar*M; % G: n*n
    E=C'*Q_bar*M; % E: NP*n
    H=C'*Q_bar*C+R_bar; % NP*NP
 J=(D'*Q_bar*C)';
 L=E*x_k+J;
 U = U_init*ones(N*p,1); % NP x 1
%  options = optimoptions('quadprog', 'Algorithm', 'active-set');
%  U_k = quadprog(H,L, [], [], [], [], 0*ones(5,1), 1100*ones(5,1), 100*ones(5,1), options);
    % 梯度下降法求解最优二次规划问题
    G=size(U,1);
    S=zeros(G*maxIterations,1);
    for i = 1:maxIterations
        % 计算目标函数的梯度
        gradient = 2*H*U + 2*L;
        % 更新变量 U，并保持在 [0, 1100] 范围内
        U = U - learningRate * gradient;
        U = max(U, 0);
        U = min(U, 1100);
        O=(i-1)*maxIterations+(1:maxIterations);
        S(O,1)=U;
    end

 u_k = S(1:p,1); % 取第一个结果
end
